simulink model "DEBUG"  (R2021a)
settings: Solver=FixedStepAuto  StartTime=0.0  StopTime=10.0  FixedStep=0.05  RelTol=1e-3
InitFcn:
  | port = 19999;
  | InitSim;
undefined symbols (not defined in the file): clientID, GetObjectPosition, PosLib, vrep
libraries: roblocks x3, JointLib x1
settings Model: Creator=Harry  LastModifiedBy=Harry

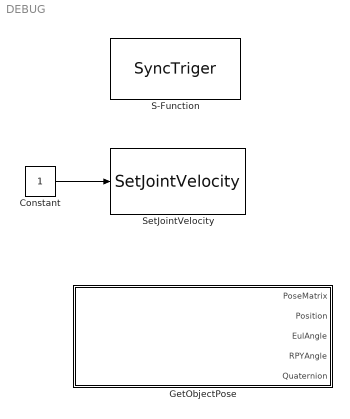
== system DEBUG ==
  Constant : Constant
  GetObjectPose : Subsystem  AncestorBlock=PosLib/GetObjectPosition  mask{object_name='L1', relative_object_name='world'}
      mask prompts: object_name "Object name:"; relative_object_name "Relative name:"
      mask DialogControl DescGroupVar Prompt: Instructions
      mask DialogControl DescTextVar Prompt: Relative Object: 'world' means relative to world frame, 'parent' means  relative to parent frame, and you can input other object name.
      mask Display:
      | port_label('output',1,'pose matrix(4*4)')
      | port_label('output',2,'position(x,y,z)')
      | port_label('output',3,'euler angle(ZYZ)')
      | port_label('output',4,'RPY angle')
      | port_label('output',5,'Quaternion')
      | 
      | if ischar(object_name)
      |     color('black');
      |     x=sprintf('GetObjectPose\n\n(%s relative to %s)',object_name,relative_object_name);
      |     disp(x);
      | else
      |     color('red');
      |     disp('Input Error');
      | end
  S-Function : S-Function  FunctionName=SyncTriger  Parameters=vrep,clientID  SFunctionDeploymentMode=off  EnableBusSupport=off
      mask Display:
      | disp('Sync triger');
      | 
      | 
      | color('red')
      | text(5,8,'VrepSim V0.1')
  SetJointVelocity : JointLib/SetJointVelocity  joint_name='Revolute_joint1'  is_use_radian=on
  wires:
  Constant/1 -> SetJointVelocity/1

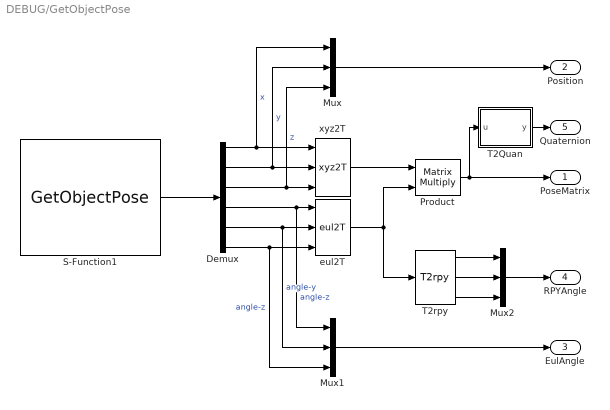
== system DEBUG/GetObjectPose ==
  Demux : Demux  Outputs=6
  Mux : Mux  Inputs=3
  Mux1 : Mux  Inputs=3
  Mux2 : Mux  Inputs=3
  Product : Product  Multiplication=Matrix(*)
  S-Function1 : S-Function  FunctionName=GetObjectPose  Parameters=vrep,clientID,object_name,relative_object_name  SFunctionDeploymentMode=off  EnableBusSupport=off
  T2Quan : MATLAB Function  TreatAsAtomicUnit=on
  T2rpy : roblocks/Toolbox/T2rpy  sequence=ZYX  degrees=off
      settings: SourceProductName=roblocks
  eul2T : roblocks/Toolbox/eul2T  degrees=off
      settings: SourceProductName=roblocks
  xyz2T : roblocks/Toolbox/xyz2T
      settings: SourceProductName=roblocks
  PoseMatrix : Outport
  Position : Outport  Port=2
  EulAngle : Outport  Port=3
  RPYAngle : Outport  Port=4
  Quaternion : Outport  Port=5
  wires:
  S-Function1/1 -> Demux/1
  Demux/1 -> Mux/1, xyz2T/1  "x"
  Demux/2 -> Mux/2, xyz2T/2  "y"
  Demux/3 -> Mux/3, xyz2T/3  "z"
  Demux/4 -> Mux1/1, eul2T/1  "angle-z"
  Demux/5 -> Mux1/2, eul2T/2  "angle-y"
  Demux/6 -> Mux1/3, eul2T/3  "angle-z"
  xyz2T/1 -> Product/1
  eul2T/1 -> T2rpy/1, Product/2
  Product/1 -> T2Quan/1(u), PoseMatrix/1
  Mux/1 -> Position/1
  Mux1/1 -> EulAngle/1
  T2rpy/1 -> Mux2/1
  T2rpy/2 -> Mux2/2
  T2rpy/3 -> Mux2/3
  Mux2/1 -> RPYAngle/1
  T2Quan/1(y) -> Quaternion/1

== matlab function DEBUG/GetObjectPose/T2Quan ==
  data: u input; y output
function y = fcn(u)
    q0 = 0.5*sqrt(1+u(1,1)+u(2,2)+u(3,3));
    q1 = (u(3,2)-u(2,3))/(4*q0);
    q2 = (u(1,3)-u(3,1))/(4*q0);
    q3 = (u(2,1)-u(1,2))/(4*q0);
    y = [q0,q1,q2,q3];
end
